simulink model "schemat_zlinearyzowany"  (R2022a)
settings: Solver=VariableStepAuto  StartTime=0.0  StopTime=50  RelTol=1e-3
values from neighbouring files (symbols this model uses):
  K = 3    [dane.m]    (also in k_stat.m = (111*ul)/50 - (171*ul.^2)/100 - (12*ul.^3)/5 + 117/100; untitled.m)
  L1 = 0.39    [dane.m]    (also in untitled.m)
  L2 = 0.37    [dane.m]    (also in untitled.m)
  L3 = -0.19    [dane.m]    (also in untitled.m)
  L4 = -0.2    [dane.m]    (also in untitled.m)
  T1 = 6    [dane.m]    (also in untitled.m)
  T2 = 7    [dane.m]    (also in untitled.m)
  Tp = 1    [dane.m]    (also in untitled.m)
  ul = -1:0.1:1    [k_stat.m]    (also in wykresy.m = -0.5)
settings Model: Creator=danie  LastModifiedBy=danie

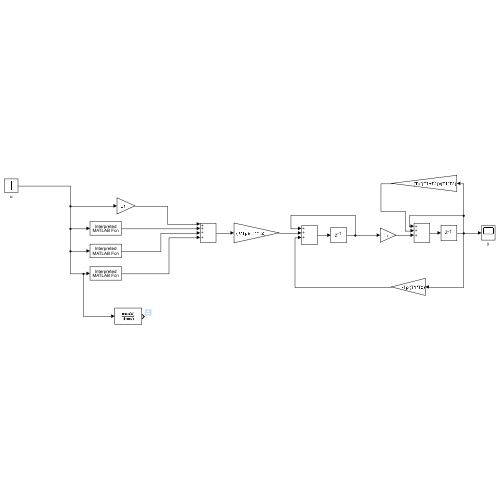
[thumbnail: Simulink's stored preview of the top-level diagram]
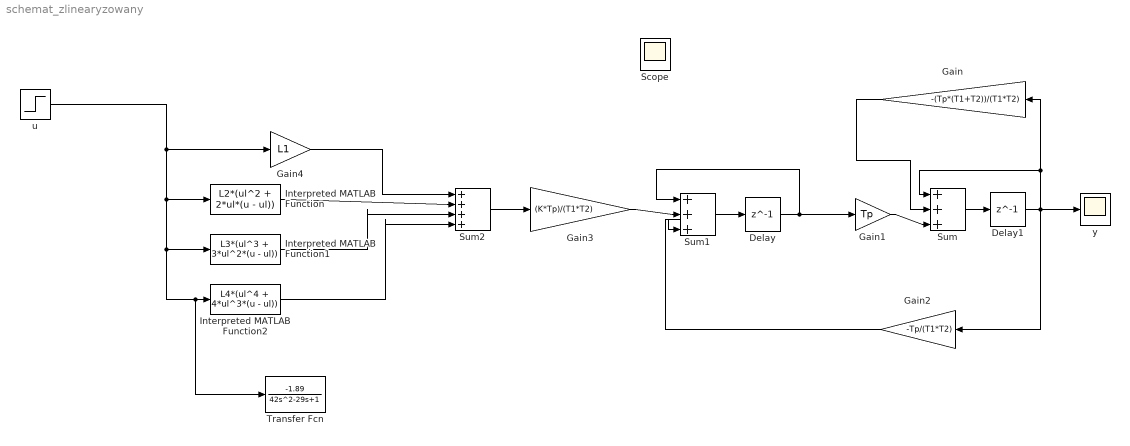
== system schemat_zlinearyzowany ==
  Delay : Delay  DelayLength=1  InitialCondition=0  SampleTime=Tp
  Delay1 : Delay  DelayLength=1  InitialCondition=0  SampleTime=Tp
  Gain : Gain  Gain=-(Tp*(T1+T2))/(T1*T2)
  Gain1 : Gain  Gain=Tp
  Gain2 : Gain  Gain=-Tp/(T1*T2)
  Gain3 : Gain  Gain=(K*Tp)/(T1*T2)
  Gain4 : Gain  Gain=L1
  Interpreted MATLAB Function : MATLABFcn  MATLABFcn=L2*(ul^2 + 2*ul*(u - ul))
  Interpreted MATLAB Function1 : MATLABFcn  MATLABFcn=L3*(ul^3 + 3*ul^2*(u - ul))
  Interpreted MATLAB Function2 : MATLABFcn  MATLABFcn=L4*(ul^4 + 4*ul^3*(u - ul))
  Sum : Sum  Inputs=+++|
  Sum1 : Sum  Inputs=+++|
  Sum2 : Sum  Inputs=++++|
  Transfer Fcn : TransferFcn  Numerator=[-1.89]  Denominator=[42 -29 1]
  u : Step  SampleTime=0
  y : Scope
  Scope : Scope
  wires:
  Delay/1 -> Sum1/1, Gain1/1
  Sum/1 -> Delay1/1
  Delay1/1 -> Gain2/1, y/1, Gain/1, Sum/1
  Gain/1 -> Sum/2
  Gain1/1 -> Sum/3
  Sum1/1 -> Delay/1
  Gain2/1 -> Sum1/3
  Gain3/1 -> Sum1/2
  u/1 -> Gain4/1, Interpreted MATLAB Function1/1, Transfer Fcn/1, Interpreted MATLAB Function2/1, Interpreted MATLAB Function/1
  Sum2/1 -> Gain3/1
  Interpreted MATLAB Function/1 -> Sum2/2
  Gain4/1 -> Sum2/1
  Interpreted MATLAB Function1/1 -> Sum2/3
  Interpreted MATLAB Function2/1 -> Sum2/4
